simulink model "WT_GC"  (R2018a)
settings: Solver=ode5  StartTime=0.0  StopTime=8  FixedStep=Ts_phy  RelTol=1e-3  EnableMultiTasking=on
values from neighbouring files (symbols this model uses):
  col = {}    [Electrical_model_settings.m]    (also in WT_GC_Script.m)
  systemBase = {}    [Electrical_model_settings.m]    (also in WT_GC_Script.m)
  Ts_phy = 1/10000    (= 0.0001)    [Electrical_model_settings.m]    (also in WT_GC_Script.m)
  Ts_sim = Ts_phy    (= 0.0001)    [WT_GC_Script.m]
  wt1 = {}    [Electrical_model_settings.m]    (also in WT_GC_Script.m)
undefined symbols (not defined in the file or in its folder): D1, Delta
libraries: pwrsysBasic x42, powerlib x16, pwrsysVICtrl x12, pwrsysVSrc x3, pwrsysTransf x3, pwrsysVSrc_202301 x2
settings Model: Creator=daniemot  LastModifiedBy=daniemot
settings OptimizationCC: LifeSpan=inf
settings DebuggingCC: SFUnexpectedBacktrackingDiag=warning  SFNoUnconditionalDefaultTransitionDiag=warning  SFExecutionAtInitializationDiag=none
settings CodeAppCC: StateflowObjectComments=on
settings GRTTargetCC: TargetLangStandard=C89/C90 (ANSI)  GeneratePreprocessorConditionals=Disable all
settings ConfigComp: CovMetricSettings=dw  CovHtmlReporting=on  CovSaveCumulativeToWorkspaceVar=on  CovSaveSingleToWorkspaceVar=on  CovExternalEMLEnable=off
settings SimscapeCC: SimscapeNormalizeSystem=off

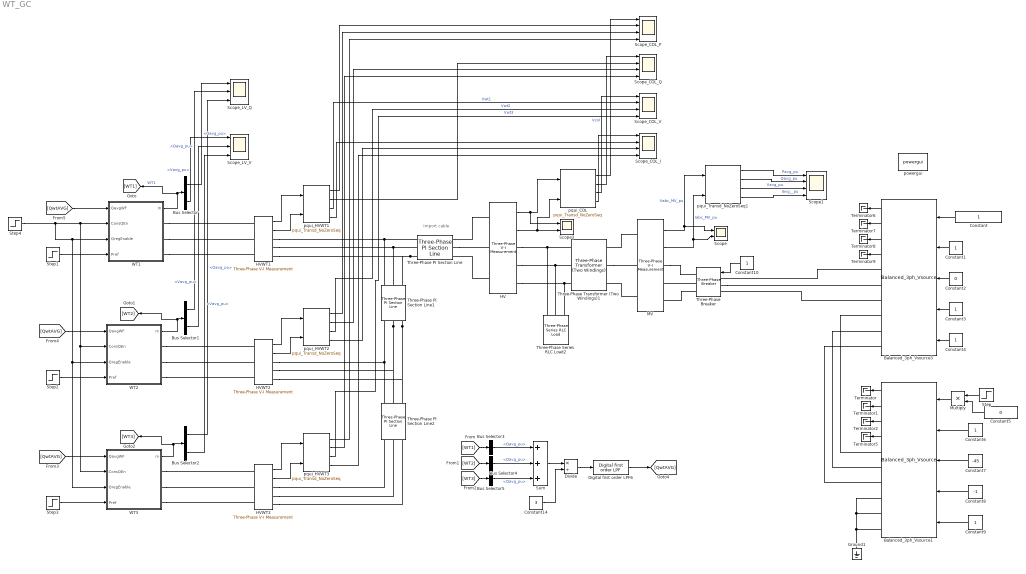
== system WT_GC ==
  note: Import cable
  Balanced_3ph_Vsource1 : pwrsysVSrc_202301/Balanced_3ph_Vsource  BaseAmp=sm.Vn_phase_peak  fn=sm.fn  AmpIni=0  SeqIni=-1  AngIni=0  FIni=sm.fn  HarmIni=1
  Balanced_3ph_Vsource3 : pwrsysVSrc_202301/Balanced_3ph_Vsource  BaseAmp=sm.Vn_phase_peak  fn=sm.fn  AmpIni=sm.Vn_phase_peak  SeqIni=1  AngIni=sm.phaseInitial  FIni=sm.initialSpeed  HarmIni=1
  Bus Selector : BusSelector  OutputSignals=Qavg_pu,Vavg_pu
  Bus Selector1 : BusSelector  OutputSignals=Qavg_pu,Vavg_pu
  Bus Selector2 : BusSelector  OutputSignals=Qavg_pu,Vavg_pu
  Bus Selector3 : BusSelector  OutputSignals=Qavg_pu
  Bus Selector4 : BusSelector  OutputSignals=Qavg_pu
  Bus Selector5 : BusSelector  OutputSignals=Qavg_pu
  Constant{,1,3..4,6,9..10} (7 alike) : Constant
  Constant14 : Constant  Value=3
  Constant2 : Constant  Value=0
  Constant5 : Constant  Value=0
  Constant7 : Constant  Value=-45
  Constant8 : Constant  Value=-1
  Digital first order LPF6 : pwrsysBasic/Digital first order LPF  Ts=wt1.Ts_control  fcutout=1
      settings: SourceProductName=NTNU Power Systems
  Divide : Product  Inputs=*/
  Ground1 : powerlib/Elements/Ground  LConnTagsString=a
  HV : powerlib/Measurements/Three-Phase V-I Measurement  VoltageMeasurement=phase-to-ground  SetLabelV=off  LabelV=vgrid  Vpu=off  VpuLL=off  CurrentMeasurement=yes  SetLabelI=off  LabelI=igrid  Ipu=off  Pbase=sn  Vbase=uab  OutputType=Complex  PhasorSimulation=off  PSBequivalent=0
  HVWT1 : powerlib/Measurements/Three-Phase V-I Measurement  VoltageMeasurement=phase-to-ground  SetLabelV=off  LabelV=vgrid  Vpu=off  VpuLL=off  CurrentMeasurement=yes  SetLabelI=off  LabelI=igrid  Ipu=off  Pbase=sn  Vbase=uab  OutputType=Complex  PhasorSimulation=off  PSBequivalent=0
  HVWT2 : powerlib/Measurements/Three-Phase V-I Measurement  VoltageMeasurement=phase-to-ground  SetLabelV=off  LabelV=vgrid  Vpu=off  VpuLL=off  CurrentMeasurement=yes  SetLabelI=off  LabelI=igrid  Ipu=off  Pbase=sn  Vbase=uab  OutputType=Complex  PhasorSimulation=off  PSBequivalent=0
  HVWT3 : powerlib/Measurements/Three-Phase V-I Measurement  VoltageMeasurement=phase-to-ground  SetLabelV=off  LabelV=vgrid  Vpu=off  VpuLL=off  CurrentMeasurement=yes  SetLabelI=off  LabelI=igrid  Ipu=off  Pbase=sn  Vbase=uab  OutputType=Complex  PhasorSimulation=off  PSBequivalent=0
  MV : powerlib/Measurements/Three-Phase V-I Measurement  VoltageMeasurement=phase-to-ground  SetLabelV=off  LabelV=vgrid  Vpu=off  VpuLL=off  CurrentMeasurement=yes  SetLabelI=off  LabelI=igrid  Ipu=off  Pbase=sn  Vbase=uab  OutputType=Complex  PhasorSimulation=off  PSBequivalent=0
  Multiply : Product
  Scope : Scope  NumInputPorts=2
  Scope1 : Scope  NumInputPorts=4
  Scope3 : Scope  NumInputPorts=2
  Scope_COL_I : Scope  NumInputPorts=4
  Scope_COL_P : Scope  NumInputPorts=4
  Scope_COL_Q : Scope  NumInputPorts=4
  Scope_COL_V : Scope  NumInputPorts=4
  Scope_LV_Q : Scope  NumInputPorts=3
  Scope_LV_V : Scope  NumInputPorts=3
  Step : Step  Time=0.1  SampleTime=0
  Step1 : Step  Time=wt1.DCVCont.Start+2.8  After=0.8  SampleTime=0
  Step2 : Step  Time=wt1.DCVCont.Start+1.8  After=0.8  SampleTime=0
  Step3 : Step  Time=wt1.DCVCont.Start+0.8  After=0.8  SampleTime=0
  Step4 : Step  Time=5  SampleTime=0
  Sum : Sum  Inputs=+++
  Terminator{,1..2,5..9} (8 alike) : Terminator
  Three-Phase PI Section Line : powerlib/Elements/Three-Phase PI Section Line  LConnTagsString=a|b|c  RConnTagsString=A|B|C  Frequency=systemBase.fn  Resistances=[ col.Cable.Rpos col.Cable.Rzero]  Inductances=[ col.Cable.Lpos col.Cable.Lzero]  Capacitances=[col.Cable.Cpos col.Cable.Czero]  Length=col.Cable.Limport
      settings: SourceProductName=Simscape Power Systems
  Three-Phase PI Section Line1 : powerlib/Elements/Three-Phase PI Section Line  LConnTagsString=a|b|c  RConnTagsString=A|B|C  Frequency=systemBase.fn  Resistances=[ col.Cable.Rpos col.Cable.Rzero]  Inductances=[ col.Cable.Lpos col.Cable.Lzero]  Capacitances=[col.Cable.Cpos col.Cable.Czero]  Length=col.Cable.LinterWT
      settings: SourceProductName=Simscape Power Systems
  Three-Phase PI Section Line2 : powerlib/Elements/Three-Phase PI Section Line  LConnTagsString=a|b|c  RConnTagsString=A|B|C  Frequency=systemBase.fn  Resistances=[ col.Cable.Rpos col.Cable.Rzero]  Inductances=[ col.Cable.Lpos col.Cable.Lzero]  Capacitances=[col.Cable.Cpos col.Cable.Czero]  Length=col.Cable.LinterWT
      settings: SourceProductName=Simscape Power Systems
  Three-Phase Series RLC Load2 : powerlib/Elements/Three-Phase Series RLC Load  LConnTagsString=A|B|C  Configuration=Y (grounded)  NominalVoltage=systemBase.Vn  Vabc=[1e3 1e3 1e3]  Vabcp=[1e3 1e3 1e3]  NominalFrequency=systemBase.fn  UnbalancedPower=off  ActivePower=100  InductivePower=0  CapacitivePower=0  Pabc=[10e3 9e3 11e3]  QLabc=[100 90 110]  QCabc=[100 90 110]  Pabcp=[10e3 9e3 11e3]  QLabcp=[100 90 110]  QCabcp=[100 90 110]  Measurements=None  LoadType=constant Z
  Three-Phase Transformer (Two Windings)1 : powerlib/Elements/Three-Phase Transformer (Two Windings)  Winding1Connection=Delta (D1)  Winding2Connection=Y  CoreType=Three-limb core (core-type)  SetSaturation=off  Hysteresis=off  DataFile='hysteresis'  SetInitialFlux=off  Measurements=None  UNITS=pu  NominalPower=[ col.Sn , systemBase.fn ]  Winding1=[ systemBase.Vn , col.Trafo.rsc/2 , col.Trafo.xsc/2 ]  Winding2=[ col.Un , col.Trafo.rsc/2 , col.Trafo.xsc/2 ]  Rm=500  Lm=500  L0=0.5  Saturation=[ 0,0 ; 0.0024,1.2 ; 1.0,1.52 ]  InitialFluxes=[ 0.8 , -0.8 , 0.7 ]  MoreParameters=off  BreakLoop=off  DataType=off  TransfoNumber=1
  Three-Phase Breaker : powerlib/Elements/Three-Phase Breaker  InitialState=closed  SwitchA=on  SwitchB=on  SwitchC=on  SwitchTimes="[1/60  5/60]"  External=on  BreakerResistance=0.01  SnubberResistance=1e6  SnubberCapacitance=1e9  Measurements=None
  WT1 : Subsystem
  WT2 : Subsystem
  WT3 : Subsystem
  powergui : powerlib/powergui  Priority=1  SimulationMode=Discrete  SampleTime=max(Ts_phy,Ts_sim)  frequency=60  Iterations=50  frequencyindice=0  Pbase=100e6  ErrMax=1e-4  UnitsV=kV  UnitsW=MW  buscounter=0  FunctionMessages=off  echomessages=off  EnableUseOfTLC=off  CurrentSourceSwitches=off  DisableSnubberDevices=off  DisableRonSwitches=off  DisableVfSwitches=off  DisplayEquations=off  SolverType=Tustin/Backward Euler (TBE)  Interpol=off  ExternalGateDelay=off  methode=off  Ts=100  x0status=blocks  SPID=off  SwTol=0  HookPort=off  RestoreLinks=warning  ResistiveCurrentMeasurement=off  Frange=[0:2:500]  Ylog=off  Xlog=on  ShowGrid=off  save=off  variable=ZData  structure=0  ZoomFFT=off  StartTime=0.0  cycles=1  DisplayStyle=1  fundamental=60  FreqAxis=off  MaxFrequency=1000  frequencyindicesteady=1  RmsSteady=1  display=off
  pqui_COL : pwrsysBasic/pqui_Transd_NoZeroSeq  Sn=col.Sn  Uanp=col.Uanp  Iap=col.Iap
      settings: SourceProductName=NTNU Power Systems
  pqui_HVWT1 : pwrsysBasic/pqui_Transd_NoZeroSeq  Sn=wt1.Sn  Uanp=col.Uanp  Iap=wt1.Iap*(wt1.Un/col.Un)
      settings: SourceProductName=NTNU Power Systems
  pqui_HVWT2 : pwrsysBasic/pqui_Transd_NoZeroSeq  Sn=wt1.Sn  Uanp=col.Uanp  Iap=wt1.Iap*(wt1.Un/col.Un)
      settings: SourceProductName=NTNU Power Systems
  pqui_HVWT3 : pwrsysBasic/pqui_Transd_NoZeroSeq  Sn=wt1.Sn  Uanp=col.Uanp  Iap=wt1.Iap*(wt1.Un/col.Un)
      settings: SourceProductName=NTNU Power Systems
  pqui_Transd_NoZeroSeq1 : pwrsysBasic/pqui_Transd_NoZeroSeq  Sn=col.Sn  Uanp=systemBase.Vn_phase*sqrt(2)  Iap=col.Iap*(col.Un/systemBase.Vn_phase)
      settings: SourceProductName=NTNU Power Systems
  wires:
  Constant/1 -> Balanced_3ph_Vsource3/1
  Balanced_3ph_Vsource3/3 -> Terminator8/1
  Balanced_3ph_Vsource1/4 -> Terminator5/1
  Step/1 -> Multiply/1
  Balanced_3ph_Vsource3/4 -> Terminator9/1
  Balanced_3ph_Vsource3/1 -> Terminator6/1
  Balanced_3ph_Vsource1/3 -> Terminator2/1
  Balanced_3ph_Vsource3/2 -> Terminator7/1
  Constant9/1 -> Balanced_3ph_Vsource1/5
  Constant2/1 -> Balanced_3ph_Vsource3/3
  Constant7/1 -> Balanced_3ph_Vsource1/3
  Constant5/1 -> Multiply/2
  Multiply/1 -> Balanced_3ph_Vsource1/1
  Constant8/1 -> Balanced_3ph_Vsource1/4
  Balanced_3ph_Vsource1/1 -> Terminator/1
  Balanced_3ph_Vsource1/2 -> Terminator1/1
  Constant3/1 -> Balanced_3ph_Vsource3/4
  Constant6/1 -> Balanced_3ph_Vsource1/2
  Constant4/1 -> Balanced_3ph_Vsource3/5
  Constant1/1 -> Balanced_3ph_Vsource3/2
  Constant10/1 -> Three-Phase Breaker/1
  MV/2 -> Scope/2, pqui_Transd_NoZeroSeq1/2  "Iabc_MV_pu"
  pqui_Transd_NoZeroSeq1/1 -> Scope1/1  "Pavg_pu"
  MV/1 -> Scope/1, pqui_Transd_NoZeroSeq1/1  "Vabc_MV_pu"
  pqui_Transd_NoZeroSeq1/3 -> Scope1/3  "Vavg_pu"
  pqui_Transd_NoZeroSeq1/2 -> Scope1/2  "Qavg_pu"
  pqui_Transd_NoZeroSeq1/4 -> Scope1/4  "Iavg__pu"
  [QwtAVG] -> WT1/1(QavgWF)
  HV/1 -> Scope3/1, pqui_COL/1
  HV/2 -> Scope3/2, pqui_COL/2
  pqui_COL/1 -> Scope_COL_P/1
  pqui_COL/2 -> Scope_COL_Q/1
  pqui_COL/3 -> Scope_COL_V/1  "Vcol"
  Step1/1 -> WT1/4(Pref)
  WT2/1(m) -> [WT2], Bus Selector1/1
  WT3/1(m) -> [WT3], Bus Selector2/1
  WT1/1(m) -> [WT1], Bus Selector/1  "WT1"
  HVWT1/2 -> pqui_HVWT1/2
  HVWT1/1 -> pqui_HVWT1/1
  pqui_HVWT1/3 -> Scope_COL_V/2  "Vwt1"
  HVWT2/1 -> pqui_HVWT2/1
  HVWT2/2 -> pqui_HVWT2/2
  HVWT3/1 -> pqui_HVWT3/1
  HVWT3/2 -> pqui_HVWT3/2
  pqui_HVWT3/3 -> Scope_COL_V/4  "Vwt3"
  pqui_HVWT2/3 -> Scope_COL_V/3  "Vwt2"
  pqui_HVWT1/2 -> Scope_COL_Q/2
  pqui_HVWT2/2 -> Scope_COL_Q/3
  pqui_HVWT3/2 -> Scope_COL_Q/4
  pqui_HVWT1/1 -> Scope_COL_P/2
  pqui_HVWT2/1 -> Scope_COL_P/3
  pqui_HVWT3/1 -> Scope_COL_P/4
  pqui_COL/4 -> Scope_COL_I/1
  pqui_HVWT1/4 -> Scope_COL_I/2
  pqui_HVWT2/4 -> Scope_COL_I/3
  pqui_HVWT3/4 -> Scope_COL_I/4
  Bus Selector/1 -> Scope_LV_Q/1  "<Qavg_pu>"
  Bus Selector1/1 -> Scope_LV_Q/2  "<Qavg_pu>"
  Bus Selector2/1 -> Scope_LV_Q/3  "<Qavg_pu>"
  Bus Selector/2 -> Scope_LV_V/1  "<Vavg_pu>"
  Bus Selector1/2 -> Scope_LV_V/2  "<Vavg_pu>"
  Bus Selector2/2 -> Scope_LV_V/3  "<Vavg_pu>"
  Step4/1 -> WT2/3(QregEnable), WT3/3(QregEnable), WT1/3(QregEnable), WT3/2(ConsQEn), WT2/2(ConsQEn), WT1/2(ConsQEn)
  Step2/1 -> WT2/4(Pref)
  Step3/1 -> WT3/4(Pref)
  [WT1] -> Bus Selector3/1
  [WT2] -> Bus Selector4/1
  [WT3] -> Bus Selector5/1
  Bus Selector3/1 -> Sum/1  "<Qavg_pu>"
  Bus Selector4/1 -> Sum/2  "<Qavg_pu>"
  Bus Selector5/1 -> Sum/3  "<Qavg_pu>"
  Sum/1 -> Divide/1
  Constant14/1 -> Divide/2
  Divide/1 -> Digital first order LPF6/1
  Digital first order LPF6/1 -> [QwtAVG]
  [QwtAVG] -> WT3/1(QavgWF)
  [QwtAVG] -> WT2/1(QavgWF)
  connections:
  Balanced_3ph_Vsource1/RConn4 -- Balanced_3ph_Vsource1/RConn6 -- Ground1/LConn1 -- Balanced_3ph_Vsource1/RConn5
  Balanced_3ph_Vsource1/RConn1 -- Balanced_3ph_Vsource3/RConn4
  Balanced_3ph_Vsource1/RConn2 -- Balanced_3ph_Vsource3/RConn5
  Balanced_3ph_Vsource1/RConn3 -- Balanced_3ph_Vsource3/RConn6
  MV/RConn1 -- Three-Phase Breaker/RConn1
  Three-Phase Breaker/RConn2 -- MV/RConn2
  Three-Phase Breaker/RConn3 -- MV/RConn3
  Three-Phase Breaker/LConn2 -- Balanced_3ph_Vsource3/RConn2
  Balanced_3ph_Vsource3/RConn1 -- Three-Phase Breaker/LConn1
  Balanced_3ph_Vsource3/RConn3 -- Three-Phase Breaker/LConn3
  Three-Phase Transformer (Two Windings)1/LConn2 -- MV/LConn2
  MV/LConn1 -- Three-Phase Transformer (Two Windings)1/LConn1
  MV/LConn3 -- Three-Phase Transformer (Two Windings)1/LConn3
  Three-Phase Series RLC Load2/LConn1 -- HV/RConn1 -- Three-Phase Transformer (Two Windings)1/RConn1
  Three-Phase Transformer (Two Windings)1/RConn2 -- HV/RConn2 -- Three-Phase Series RLC Load2/LConn2
  Three-Phase Transformer (Two Windings)1/RConn3 -- HV/RConn3 -- Three-Phase Series RLC Load2/LConn3
  Three-Phase PI Section Line1/LConn1 -- HVWT1/RConn1 -- Three-Phase PI Section Line/LConn1
  Three-Phase PI Section Line/LConn3 -- HVWT1/RConn3 -- Three-Phase PI Section Line1/LConn3
  Three-Phase PI Section Line1/LConn2 -- HVWT1/RConn2 -- Three-Phase PI Section Line/LConn2
  HV/LConn1 -- Three-Phase PI Section Line/RConn1
  Three-Phase PI Section Line/RConn2 -- HV/LConn2
  HV/LConn3 -- Three-Phase PI Section Line/RConn3
  Three-Phase PI Section Line2/LConn1 -- HVWT2/RConn1 -- Three-Phase PI Section Line1/RConn1
  Three-Phase PI Section Line1/RConn2 -- Three-Phase PI Section Line2/LConn2 -- HVWT2/RConn2
  Three-Phase PI Section Line1/RConn3 -- Three-Phase PI Section Line2/LConn3 -- HVWT2/RConn3
  WT1/RConn1 -- HVWT1/LConn1
  WT1/RConn2 -- HVWT1/LConn2
  WT1/RConn3 -- HVWT1/LConn3
  WT2/RConn1 -- HVWT2/LConn1
  WT2/RConn2 -- HVWT2/LConn2
  WT2/RConn3 -- HVWT2/LConn3
  WT3/RConn1 -- HVWT3/LConn1
  WT3/RConn2 -- HVWT3/LConn2
  WT3/RConn3 -- HVWT3/LConn3
  HVWT3/RConn1 -- Three-Phase PI Section Line2/RConn1
  HVWT3/RConn2 -- Three-Phase PI Section Line2/RConn2
  HVWT3/RConn3 -- Three-Phase PI Section Line2/RConn3

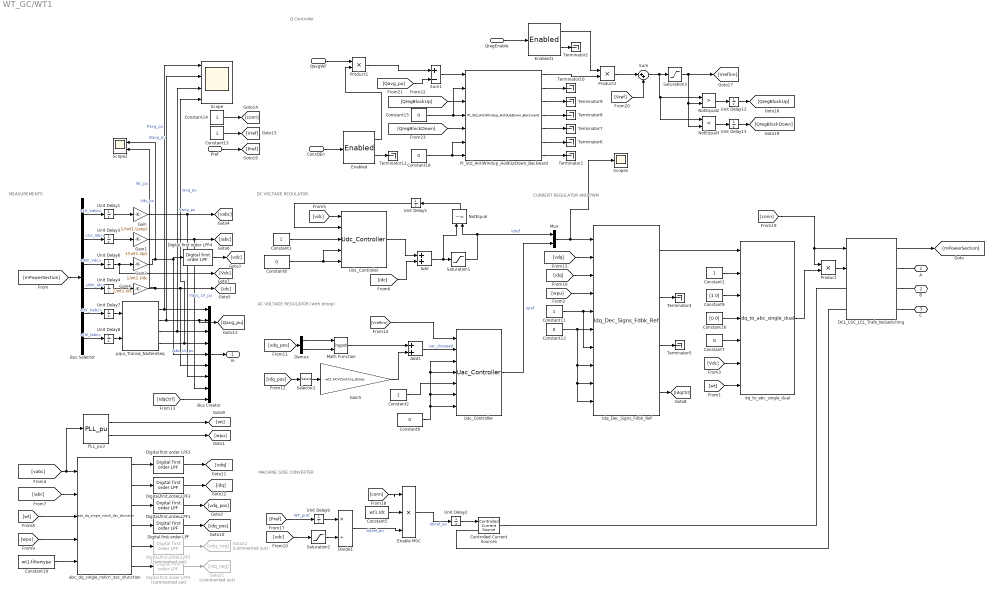
== system WT_GC/WT1 ==
  note: MEASUREMENTS
  note: MACHINE SIDE CONVERTER
  note: AC VOLTAGE REGULATOR (with droop)
  note: DC VOLTAGE REGULATOR
  note: CURRENT REGULATOR AND PWM
  note: Q Controller
  QavgWF : Inport
  ConsQEn : Inport  Port=2
  QregEnable : Inport  Port=3
  Pref : Inport  Port=4
  Add : Sum
  Add1 : Sum
  Bus Creator : BusCreator  Inputs=9
  Bus Selector : BusSelector  OutputSignals=LV_Vabc,LV_Iabc,INV_Vdc,INV_Idc,HV_Vabc,HV_Iabc
  Constant{1..3,11} (4 alike) : Constant  SampleTime=wt1.Ts_control
  Constant10 : Constant  Value=wt1.filtertype  SampleTime=wt1.Ts_control
  Constant{6..8,12} (4 alike) : Constant  Value=0  SampleTime=wt1.Ts_control
  Constant13 : Constant
  Constant14 : Constant
  Constant15 : Constant  Value=0
  Constant16 : Constant  Value=[0 0]  SampleTime=wt1.Ts_control
  Constant18 : Constant  Value=0
  Constant5 : Constant  Value=wt1.Idc  SampleTime=wt1.Ts_control
  Constant9 : Constant  Value=[1 0]  SampleTime=wt1.Ts_control
  Controlled Current Source1 : powerlib/Electrical Sources/Controlled Current Source  Initialize=on  Source_Type=DC  Amplitude=0  Phase=0  Frequency=50  Measurements=None
  DCL_LSC_LCL_Trafo_NoSwitching : pwrsysVSrc/DCL_LSC_LCL_Trafo_NoSwitching  Sn=wt1.Sn  fn=systemBase.fn  Uhv_ab=col.Un  Uab=wt1.Un  lf2=wt1.LCL.l2  rf2=wt1.LCL.r2  Lf1=wt1.LCL.L1  Rf1=wt1.LCL.R1  Cf=wt1.LCL.Cf  Rc=wt1.LCL.Rf  Cdc=wt1.Cdc  Udc0=wt1.Udc  Tsm=wt1.Ts_control  Tstart=wt1.DCVCont.Start
      settings: SourceProductName=NTNU Power Systems
  Demux : Demux  Outputs=2
  Digital first order LPF{,1..4} (5 alike) : pwrsysBasic/Digital first order LPF  Ts=wt1.Ts_control  fcutout=wt1.CurrCont.f_LPF_noise
      settings: SourceProductName=NTNU Power Systems
  Digital first order LPF5 : pwrsysBasic/Digital first order LPF  Commented=on  Ts=wt1.Ts_control  fcutout=wt1.CurrCont.f_LPF_noise
      settings: SourceProductName=NTNU Power Systems
  Digital first order LPF6 : pwrsysBasic/Digital first order LPF  Commented=on  Ts=wt1.Ts_control  fcutout=wt1.CurrCont.f_LPF_noise
      settings: SourceProductName=NTNU Power Systems
  Divide1 : Product  Inputs=*/
  Enable MSC : Product  Inputs=3
  Enabled : pwrsysBasic/Enabled
      settings: SourceProductName=NTNU Power Systems
  Enabled1 : pwrsysBasic/Enabled
      settings: SourceProductName=NTNU Power Systems
  Gain : Gain  Gain=1/(wt1.Uanp)
  Gain1 : Gain  Gain=1/(wt1.Iap)
  Gain2 : Gain  Gain=1/wt1.Udc
  Gain4 : Gain  Gain=1/wt1.Idc
  Gain5 : Gain  Gain=-wt1.ACVCont.kiq_droop
  Goto21 : Goto  Commented=on  GotoTag=idq_neg
  Goto22 : Goto  Commented=on  GotoTag=vdq_neg
  Idq_Dec_Signs_Fdbk_Ref : pwrsysVICtrl/Idq_Dec_Signs_Fdbk_Ref  Ts=wt1.Ts_control  fn=systemBase.fn  Kp=wt1.CurrContSingle.kp  Ti=wt1.CurrContSingle.Ti  L=wt1.CurrCont.x  PI_max=wt1.CurrCont.PImax  PI_min=wt1.CurrCont.PImin  TrafoPhaseComp=0
      settings: SourceProductName=NTNU Power Systems
  Math Function : Math  Operator=hypot  SaturateOnIntegerOverflow=on
  Mux : Mux  Inputs=2
  NotEqual : RelationalOperator  Operator=~=  OutDataTypeStr=boolean  RndMeth=Nearest
  NotEqual2 : RelationalOperator  Operator=>  OutDataTypeStr=boolean  RndMeth=Nearest
  NotEqual3 : RelationalOperator  Operator=<  OutDataTypeStr=boolean  RndMeth=Nearest
  PI_Std_AntiWindup_HoldUpDown_Backward : pwrsysBasic/PI_Std_AntiWindup_HoldUpDown_Backward  Ts=wt1.Ts_control  Kg=wt1.Qctrl.Kg  Kp=wt1.Qctrl.Kp  Ti=wt1.Qctrl.Ti  outMax=wt1.Qctrl.deltaUmaxPos  outMin=wt1.Qctrl.deltaUmaxNeg
      settings: SourceProductName=NTNU Power Systems
  PLL_pu3 : pwrsysBasic/PLL_pu  fn=systemBase.fn  Ts=wt1.Ts_control  Kp_pll=90  Ki_pll=1200  Kd_pll=0  PLL_ini=60
      settings: SourceProductName=NTNU Power Systems
  Product : Product
  Product1 : Product
  Product2 : Product
  Saturation1 : Saturate  UpperLimit=wt1.DCVCont.PImax  LowerLimit=wt1.DCVCont.PImin
  Saturation2 : Saturate  UpperLimit=1.2  LowerLimit=0.8
  Saturation3 : Saturate  UpperLimit=wt1.Qctrl.Umax  LowerLimit=wt1.Qctrl.Umin
  Scope : Scope  NumInputPorts=4
  Scope1 : Scope
  Scope2 : Scope  NumInputPorts=2
  Selector2 : Selector  IndexMode=Zero-based  InputPortWidth=2  IndexOptions=Index vector (dialog)  Indices=1  OutputSizes=1
  Sum : Sum  Inputs=|++
  Sum1 : Sum  Inputs=+-
  Terminator{1..2,4..10,12} (10 alike) : Terminator
  Uac_Controller : pwrsysVICtrl/Uac_Controller  Ts=wt1.Ts_control  Kg=wt1.ACVCont.kg  Kp=wt1.ACVCont.kp  Ti=wt1.ACVCont.Ti  PI_max=wt1.ACVCont.PImax  PI_min=wt1.ACVCont.PImin
      settings: SourceProductName=NTNU Power Systems
  Udc_Controller : pwrsysVICtrl/Udc_Controller  Ts=wt1.Ts_control  Kp=wt1.DCVContSingle.kp  Ti=wt1.DCVContSingle.Ti  PI_max=wt1.DCVCont.PImax  PI_min=wt1.DCVCont.PImin
      settings: SourceProductName=NTNU Power Systems
  Unit Delay{1,3,7..8} (4 alike) : UnitDelay  InitialCondition=[0 0 0]  SampleTime=wt1.Ts_control
  Unit Delay{2,4..5,9,12..13} (6 alike) : UnitDelay  SampleTime=wt1.Ts_control
  Unit Delay6 : UnitDelay  InitialCondition=1  SampleTime=wt1.Ts_control
  abc_dq_single_notch_dsc_sfunction : pwrsysTransf/abc_dq_single_notch_dsc_sfunction  Ts=wt1.Ts_control  fn=2*systemBase.fn  zeta=wt1.CurrCont.zeta
      settings: SourceProductName=NTNU Power Systems
  dq_to_abc_single_dual : pwrsysVICtrl/dq_to_abc_single_dual  Ts=wt1.Ts_control  Uabp=wt1.Uabp
      settings: SourceProductName=NTNU Power Systems
  pqui_Transd_NoZeroSeq : pwrsysBasic/pqui_Transd_NoZeroSeq  Sn=wt1.Sn  Uanp=col.Uanp  Iap=wt1.Iap*(wt1.Un/col.Un)
      settings: SourceProductName=NTNU Power Systems
  A : PMIOPort  Side=Right
  B : PMIOPort  Port=2  Side=Right
  C : PMIOPort  Port=3  Side=Right
  m : Outport
  wires:
  Divide1/1 -> Enable MSC/3  "Idcref_pu"
  Bus Selector/1 -> Unit Delay1/1  "<LV_Vabc>"
  [idq_pos] -> Selector2/1
  Unit Delay2/1 -> Controlled Current Source1/1
  Gain1/1 -> Bus Creator/8, [iabc]  "Iabc_LV_pu"
  Bus Selector/2 -> Unit Delay3/1  "<LV_Iabc>"
  Gain5/1 -> Add1/2
  Math Function/1 -> Add1/1
  Constant6/1 -> Uac_Controller/7, Uac_Controller/6, Uac_Controller/3, Uac_Controller/4
  Constant5/1 -> Enable MSC/2
  Add1/1 -> Uac_Controller/2  "vac_drooped"
  [mPowerSection] -> Bus Selector/1
  Enable MSC/1 -> Unit Delay2/1  "Idcref_pu"
  Gain/1 -> Bus Creator/7, [vabc]  "Vabc_LV_pu"
  Constant2/1 -> Uac_Controller/5
  Constant8/1 -> Udc_Controller/4, Udc_Controller/5
  NotEqual/1 -> Unit Delay5/1
  [vdc] -> Udc_Controller/1
  Unit Delay5/1 -> Udc_Controller/2
  Saturation1/1 -> NotEqual/2, Mux/1  "idref"
  [idc] -> Add/2
  Udc_Controller/1 -> Add/1
  Add/1 -> NotEqual/1, Saturation1/1
  Constant3/1 -> Udc_Controller/3
  [idq] -> Idq_Dec_Signs_Fdbk_Ref/3
  [Vdc] -> dq_to_abc_single_dual/6
  [wpu] -> Idq_Dec_Signs_Fdbk_Ref/4
  dq_to_abc_single_dual/1 -> Product/2
  [conn] -> Product/1, DCL_LSC_LCL_Trafo_NoSwitching/1
  Saturation2/1 -> Divide1/2
  [Pref] -> Unit Delay9/1  "WT_pref"
  [vdc] -> Saturation2/1
  [wt] -> dq_to_abc_single_dual/7
  Constant10/1 -> abc_dq_single_notch_dsc_sfunction/5
  Bus Selector/5 -> Unit Delay7/1  "<HV_Vabc>"
  Bus Selector/6 -> Unit Delay8/1  "<HV_Iabc>"
  pqui_Transd_NoZeroSeq/1 -> Scope/1, Bus Creator/1  "Pavg_pu"
  pqui_Transd_NoZeroSeq/2 -> Scope/2, [Qavg_pu], Bus Creator/2  "Qavg_pu"
  pqui_Transd_NoZeroSeq/3 -> Scope/3, Bus Creator/3  "Vavg_pu"
  pqui_Transd_NoZeroSeq/4 -> Scope/4, Bus Creator/4  "Iavg_pu"
  Bus Creator/1 -> m/1
  Bus Selector/3 -> Unit Delay6/1  "<INV_Vdc>"
  Gain2/1 -> Scope2/1, Digital first order LPF4/1, Bus Creator/5  "Vdc_pu"
  Gain4/1 -> Scope2/2, [idc], Bus Creator/6  "Idc_pu"
  Bus Selector/4 -> Unit Delay4/1  "<INV_Idc>"
  PLL_pu3/2 -> [wpu]
  PLL_pu3/1 -> [wt]
  Uac_Controller/1 -> Mux/2  "iqref"
  DCL_LSC_LCL_Trafo_NoSwitching/1 -> [mPowerSection]
  Unit Delay1/1 -> Gain/1
  Unit Delay3/1 -> Gain1/1
  Unit Delay4/1 -> Gain4/1
  Unit Delay8/1 -> pqui_Transd_NoZeroSeq/2
  Unit Delay6/1 -> [Vdc], Gain2/1
  Unit Delay7/1 -> pqui_Transd_NoZeroSeq/1
  Unit Delay9/1 -> Divide1/1
  [Vreflim] -> Uac_Controller/1
  abc_dq_single_notch_dsc_sfunction/6 -> Digital first order LPF6/1
  abc_dq_single_notch_dsc_sfunction/5 -> Digital first order LPF5/1
  Selector2/1 -> Gain5/1
  Idq_Dec_Signs_Fdbk_Ref/2 -> Terminator4/1
  [vdq] -> Idq_Dec_Signs_Fdbk_Ref/2
  Constant1/1 -> dq_to_abc_single_dual/2
  Constant7/1 -> dq_to_abc_single_dual/5
  Constant11/1 -> Idq_Dec_Signs_Fdbk_Ref/7, Idq_Dec_Signs_Fdbk_Ref/5
  Constant12/1 -> Idq_Dec_Signs_Fdbk_Ref/8, Idq_Dec_Signs_Fdbk_Ref/9, Idq_Dec_Signs_Fdbk_Ref/10, Idq_Dec_Signs_Fdbk_Ref/6
  Idq_Dec_Signs_Fdbk_Ref/3 -> Terminator5/1
  Idq_Dec_Signs_Fdbk_Ref/4 -> [IdqCtrl]
  [IdqCtrl] -> Bus Creator/9
  Idq_Dec_Signs_Fdbk_Ref/1 -> dq_to_abc_single_dual/1
  [wt] -> abc_dq_single_notch_dsc_sfunction/3
  [wpu] -> abc_dq_single_notch_dsc_sfunction/4
  abc_dq_single_notch_dsc_sfunction/1 -> Digital first order LPF2/1
  [vabc] -> abc_dq_single_notch_dsc_sfunction/1, PLL_pu3/1
  [iabc] -> abc_dq_single_notch_dsc_sfunction/2
  abc_dq_single_notch_dsc_sfunction/3 -> Digital first order LPF1/1
  abc_dq_single_notch_dsc_sfunction/4 -> Digital first order LPF/1
  abc_dq_single_notch_dsc_sfunction/2 -> Digital first order LPF3/1
  Digital first order LPF/1 -> [idq_pos]
  Digital first order LPF1/1 -> [vdq_pos]
  [vdq_pos] -> Demux/1
  Demux/1 -> Math Function/1
  Demux/2 -> Math Function/2
  Digital first order LPF2/1 -> [vdq]
  Digital first order LPF3/1 -> [idq]
  Digital first order LPF4/1 -> [vdc]
  [conn] -> Enable MSC/1
  Pref/1 -> [Pref]
  Mux/1 -> Scope1/1, Idq_Dec_Signs_Fdbk_Ref/1
  Product/1 -> DCL_LSC_LCL_Trafo_NoSwitching/2
  [Vref] -> Sum/2
  Sum/1 -> NotEqual3/1, NotEqual2/1, Saturation3/1
  Saturation3/1 -> NotEqual3/2, NotEqual2/2, [Vreflim]
  [Qavg_pu] -> Sum1/2
  ConsQEn/1 -> Enabled/1
  [QregBlockUp] -> PI_Std_AntiWindup_HoldUpDown_Backward/3
  Constant15/1 -> PI_Std_AntiWindup_HoldUpDown_Backward/2, PI_Std_AntiWindup_HoldUpDown_Backward/4
  [QregBlockDown] -> PI_Std_AntiWindup_HoldUpDown_Backward/5
  Constant18/1 -> PI_Std_AntiWindup_HoldUpDown_Backward/6, PI_Std_AntiWindup_HoldUpDown_Backward/7
  PI_Std_AntiWindup_HoldUpDown_Backward/7 -> Terminator1/1
  PI_Std_AntiWindup_HoldUpDown_Backward/6 -> Terminator6/1
  PI_Std_AntiWindup_HoldUpDown_Backward/5 -> Terminator7/1
  PI_Std_AntiWindup_HoldUpDown_Backward/4 -> Terminator8/1
  PI_Std_AntiWindup_HoldUpDown_Backward/3 -> Terminator9/1
  PI_Std_AntiWindup_HoldUpDown_Backward/2 -> Terminator10/1
  NotEqual2/1 -> Unit Delay12/1
  Unit Delay12/1 -> [QregBlockUp]
  NotEqual3/1 -> Unit Delay13/1
  Unit Delay13/1 -> [QregBlockDown]
  Product2/1 -> Sum/1
  Sum1/1 -> PI_Std_AntiWindup_HoldUpDown_Backward/1
  Enabled/2 -> Terminator12/1
  QavgWF/1 -> Product1/1
  Product1/1 -> Sum1/1
  Enabled/1 -> Product1/2
  Constant13/1 -> [Vref]
  Constant14/1 -> [conn]
  Digital first order LPF5/1 -> Goto22/1
  Digital first order LPF6/1 -> Goto21/1
  Constant9/1 -> dq_to_abc_single_dual/3
  Constant16/1 -> dq_to_abc_single_dual/4
  Enabled1/2 -> Terminator2/1
  PI_Std_AntiWindup_HoldUpDown_Backward/1 -> Product2/2
  Enabled1/1 -> Product2/1
  QregEnable/1 -> Enabled1/1
  connections:
  Controlled Current Source1/RConn1 -- DCL_LSC_LCL_Trafo_NoSwitching/LConn1
  DCL_LSC_LCL_Trafo_NoSwitching/RConn3 -- C/RConn1
  DCL_LSC_LCL_Trafo_NoSwitching/RConn1 -- A/RConn1
  DCL_LSC_LCL_Trafo_NoSwitching/RConn2 -- B/RConn1
  Controlled Current Source1/LConn1 -- DCL_LSC_LCL_Trafo_NoSwitching/LConn2

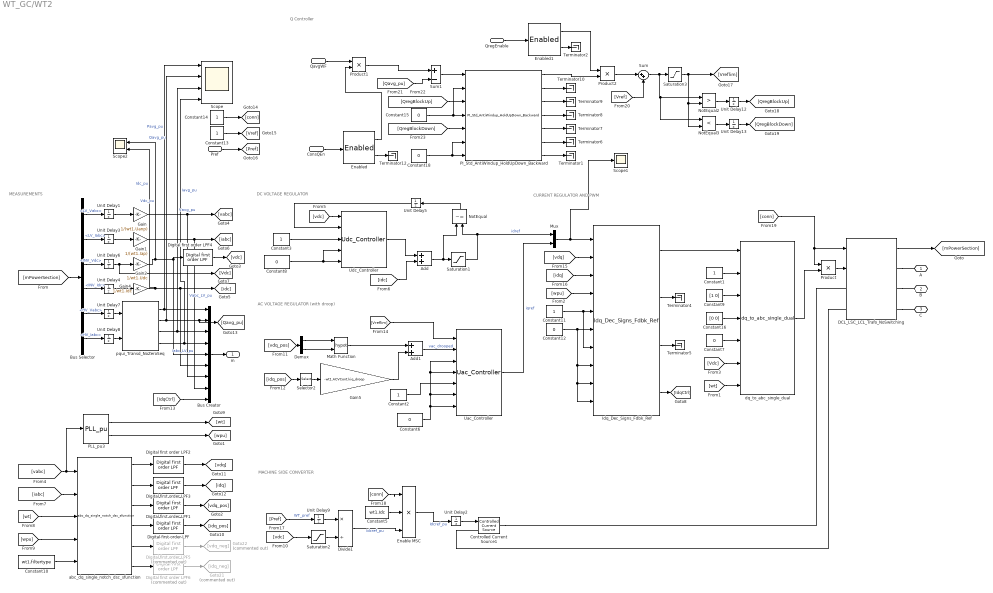
== system WT_GC/WT2 ==
  note: MEASUREMENTS
  note: MACHINE SIDE CONVERTER
  note: AC VOLTAGE REGULATOR (with droop)
  note: DC VOLTAGE REGULATOR
  note: CURRENT REGULATOR AND PWM
  note: Q Controller
  QavgWF : Inport
  ConsQEn : Inport  Port=2
  QregEnable : Inport  Port=3
  Pref : Inport  Port=4
  Add : Sum
  Add1 : Sum
  Bus Creator : BusCreator  Inputs=9
  Bus Selector : BusSelector  OutputSignals=LV_Vabc,LV_Iabc,INV_Vdc,INV_Idc,HV_Vabc,HV_Iabc
  Constant{1..3,11} (4 alike) : Constant  SampleTime=wt1.Ts_control
  Constant10 : Constant  Value=wt1.filtertype  SampleTime=wt1.Ts_control
  Constant{6..8,12} (4 alike) : Constant  Value=0  SampleTime=wt1.Ts_control
  Constant13 : Constant
  Constant14 : Constant
  Constant15 : Constant  Value=0
  Constant16 : Constant  Value=[0 0]  SampleTime=wt1.Ts_control
  Constant18 : Constant  Value=0
  Constant5 : Constant  Value=wt1.Idc  SampleTime=wt1.Ts_control
  Constant9 : Constant  Value=[1 0]  SampleTime=wt1.Ts_control
  Controlled Current Source1 : powerlib/Electrical Sources/Controlled Current Source  Initialize=on  Source_Type=DC  Amplitude=0  Phase=0  Frequency=50  Measurements=None
  DCL_LSC_LCL_Trafo_NoSwitching : pwrsysVSrc/DCL_LSC_LCL_Trafo_NoSwitching  Sn=wt1.Sn  fn=systemBase.fn  Uhv_ab=col.Un  Uab=wt1.Un  lf2=wt1.LCL.l2  rf2=wt1.LCL.r2  Lf1=wt1.LCL.L1  Rf1=wt1.LCL.R1  Cf=wt1.LCL.Cf  Rc=wt1.LCL.Rf  Cdc=wt1.Cdc  Udc0=wt1.Udc  Tsm=wt1.Ts_control  Tstart=wt1.DCVCont.Start
      settings: SourceProductName=NTNU Power Systems
  Demux : Demux  Outputs=2
  Digital first order LPF{,1..4} (5 alike) : pwrsysBasic/Digital first order LPF  Ts=wt1.Ts_control  fcutout=wt1.CurrCont.f_LPF_noise
      settings: SourceProductName=NTNU Power Systems
  Digital first order LPF5 : pwrsysBasic/Digital first order LPF  Commented=on  Ts=wt1.Ts_control  fcutout=wt1.CurrCont.f_LPF_noise
      settings: SourceProductName=NTNU Power Systems
  Digital first order LPF6 : pwrsysBasic/Digital first order LPF  Commented=on  Ts=wt1.Ts_control  fcutout=wt1.CurrCont.f_LPF_noise
      settings: SourceProductName=NTNU Power Systems
  Divide1 : Product  Inputs=*/
  Enable MSC : Product  Inputs=3
  Enabled : pwrsysBasic/Enabled
      settings: SourceProductName=NTNU Power Systems
  Enabled1 : pwrsysBasic/Enabled
      settings: SourceProductName=NTNU Power Systems
  Gain : Gain  Gain=1/(wt1.Uanp)
  Gain1 : Gain  Gain=1/(wt1.Iap)
  Gain2 : Gain  Gain=1/wt1.Udc
  Gain4 : Gain  Gain=1/wt1.Idc
  Gain5 : Gain  Gain=-wt1.ACVCont.kiq_droop
  Goto21 : Goto  Commented=on  GotoTag=idq_neg
  Goto22 : Goto  Commented=on  GotoTag=vdq_neg
  Idq_Dec_Signs_Fdbk_Ref : pwrsysVICtrl/Idq_Dec_Signs_Fdbk_Ref  Ts=wt1.Ts_control  fn=systemBase.fn  Kp=wt1.CurrContSingle.kp  Ti=wt1.CurrContSingle.Ti  L=wt1.CurrCont.x  PI_max=wt1.CurrCont.PImax  PI_min=wt1.CurrCont.PImin  TrafoPhaseComp=0
      settings: SourceProductName=NTNU Power Systems
  Math Function : Math  Operator=hypot  SaturateOnIntegerOverflow=on
  Mux : Mux  Inputs=2
  NotEqual : RelationalOperator  Operator=~=  OutDataTypeStr=boolean  RndMeth=Nearest
  NotEqual2 : RelationalOperator  Operator=>  OutDataTypeStr=boolean  RndMeth=Nearest
  NotEqual3 : RelationalOperator  Operator=<  OutDataTypeStr=boolean  RndMeth=Nearest
  PI_Std_AntiWindup_HoldUpDown_Backward : pwrsysBasic/PI_Std_AntiWindup_HoldUpDown_Backward  Ts=wt1.Ts_control  Kg=wt1.Qctrl.Kg  Kp=wt1.Qctrl.Kp  Ti=wt1.Qctrl.Ti  outMax=wt1.Qctrl.deltaUmaxPos  outMin=wt1.Qctrl.deltaUmaxNeg
      settings: SourceProductName=NTNU Power Systems
  PLL_pu3 : pwrsysBasic/PLL_pu  fn=systemBase.fn  Ts=wt1.Ts_control  Kp_pll=90  Ki_pll=1200  Kd_pll=0  PLL_ini=60
      settings: SourceProductName=NTNU Power Systems
  Product : Product
  Product1 : Product
  Product2 : Product
  Saturation1 : Saturate  UpperLimit=wt1.DCVCont.PImax  LowerLimit=wt1.DCVCont.PImin
  Saturation2 : Saturate  UpperLimit=1.2  LowerLimit=0.8
  Saturation3 : Saturate  UpperLimit=wt1.Qctrl.Umax  LowerLimit=wt1.Qctrl.Umin
  Scope : Scope  NumInputPorts=4
  Scope1 : Scope
  Scope2 : Scope  NumInputPorts=2
  Selector2 : Selector  IndexMode=Zero-based  InputPortWidth=2  IndexOptions=Index vector (dialog)  Indices=1  OutputSizes=1
  Sum : Sum  Inputs=|++
  Sum1 : Sum  Inputs=+-
  Terminator{1..2,4..10,12} (10 alike) : Terminator
  Uac_Controller : pwrsysVICtrl/Uac_Controller  Ts=wt1.Ts_control  Kg=wt1.ACVCont.kg  Kp=wt1.ACVCont.kp  Ti=wt1.ACVCont.Ti  PI_max=wt1.ACVCont.PImax  PI_min=wt1.ACVCont.PImin
      settings: SourceProductName=NTNU Power Systems
  Udc_Controller : pwrsysVICtrl/Udc_Controller  Ts=wt1.Ts_control  Kp=wt1.DCVContSingle.kp  Ti=wt1.DCVContSingle.Ti  PI_max=wt1.DCVCont.PImax  PI_min=wt1.DCVCont.PImin
      settings: SourceProductName=NTNU Power Systems
  Unit Delay{1,3,7..8} (4 alike) : UnitDelay  InitialCondition=[0 0 0]  SampleTime=wt1.Ts_control
  Unit Delay{2,4..5,9,12..13} (6 alike) : UnitDelay  SampleTime=wt1.Ts_control
  Unit Delay6 : UnitDelay  InitialCondition=1  SampleTime=wt1.Ts_control
  abc_dq_single_notch_dsc_sfunction : pwrsysTransf/abc_dq_single_notch_dsc_sfunction  Ts=wt1.Ts_control  fn=2*systemBase.fn  zeta=wt1.CurrCont.zeta
      settings: SourceProductName=NTNU Power Systems
  dq_to_abc_single_dual : pwrsysVICtrl/dq_to_abc_single_dual  Ts=wt1.Ts_control  Uabp=wt1.Uabp
      settings: SourceProductName=NTNU Power Systems
  pqui_Transd_NoZeroSeq : pwrsysBasic/pqui_Transd_NoZeroSeq  Sn=wt1.Sn  Uanp=col.Uanp  Iap=wt1.Iap*(wt1.Un/col.Un)
      settings: SourceProductName=NTNU Power Systems
  A : PMIOPort  Side=Right
  B : PMIOPort  Port=2  Side=Right
  C : PMIOPort  Port=3  Side=Right
  m : Outport
  wires:
  Divide1/1 -> Enable MSC/3  "Idcref_pu"
  Bus Selector/1 -> Unit Delay1/1  "<LV_Vabc>"
  [idq_pos] -> Selector2/1
  Unit Delay2/1 -> Controlled Current Source1/1
  Gain1/1 -> Bus Creator/8, [iabc]  "Iabc_LV_pu"
  Bus Selector/2 -> Unit Delay3/1  "<LV_Iabc>"
  Gain5/1 -> Add1/2
  Math Function/1 -> Add1/1
  Constant6/1 -> Uac_Controller/7, Uac_Controller/6, Uac_Controller/3, Uac_Controller/4
  Constant5/1 -> Enable MSC/2
  Add1/1 -> Uac_Controller/2  "vac_drooped"
  [mPowerSection] -> Bus Selector/1
  Enable MSC/1 -> Unit Delay2/1  "Idcref_pu"
  Gain/1 -> Bus Creator/7, [vabc]  "Vabc_LV_pu"
  Constant2/1 -> Uac_Controller/5
  Constant8/1 -> Udc_Controller/4, Udc_Controller/5
  NotEqual/1 -> Unit Delay5/1
  [vdc] -> Udc_Controller/1
  Unit Delay5/1 -> Udc_Controller/2
  Saturation1/1 -> NotEqual/2, Mux/1  "idref"
  [idc] -> Add/2
  Udc_Controller/1 -> Add/1
  Add/1 -> NotEqual/1, Saturation1/1
  Constant3/1 -> Udc_Controller/3
  [idq] -> Idq_Dec_Signs_Fdbk_Ref/3
  [Vdc] -> dq_to_abc_single_dual/6
  [wpu] -> Idq_Dec_Signs_Fdbk_Ref/4
  dq_to_abc_single_dual/1 -> Product/2
  [conn] -> Product/1, DCL_LSC_LCL_Trafo_NoSwitching/1
  Saturation2/1 -> Divide1/2
  [Pref] -> Unit Delay9/1  "WT_pref"
  [vdc] -> Saturation2/1
  [wt] -> dq_to_abc_single_dual/7
  Constant10/1 -> abc_dq_single_notch_dsc_sfunction/5
  Bus Selector/5 -> Unit Delay7/1  "<HV_Vabc>"
  Bus Selector/6 -> Unit Delay8/1  "<HV_Iabc>"
  pqui_Transd_NoZeroSeq/1 -> Scope/1, Bus Creator/1  "Pavg_pu"
  pqui_Transd_NoZeroSeq/2 -> Scope/2, [Qavg_pu], Bus Creator/2  "Qavg_pu"
  pqui_Transd_NoZeroSeq/3 -> Scope/3, Bus Creator/3  "Vavg_pu"
  pqui_Transd_NoZeroSeq/4 -> Scope/4, Bus Creator/4  "Iavg_pu"
  Bus Creator/1 -> m/1
  Bus Selector/3 -> Unit Delay6/1  "<INV_Vdc>"
  Gain2/1 -> Scope2/1, Digital first order LPF4/1, Bus Creator/5  "Vdc_pu"
  Gain4/1 -> Scope2/2, [idc], Bus Creator/6  "Idc_pu"
  Bus Selector/4 -> Unit Delay4/1  "<INV_Idc>"
  PLL_pu3/2 -> [wpu]
  PLL_pu3/1 -> [wt]
  Uac_Controller/1 -> Mux/2  "iqref"
  DCL_LSC_LCL_Trafo_NoSwitching/1 -> [mPowerSection]
  Unit Delay1/1 -> Gain/1
  Unit Delay3/1 -> Gain1/1
  Unit Delay4/1 -> Gain4/1
  Unit Delay8/1 -> pqui_Transd_NoZeroSeq/2
  Unit Delay6/1 -> [Vdc], Gain2/1
  Unit Delay7/1 -> pqui_Transd_NoZeroSeq/1
  Unit Delay9/1 -> Divide1/1
  [Vreflim] -> Uac_Controller/1
  abc_dq_single_notch_dsc_sfunction/6 -> Digital first order LPF6/1
  abc_dq_single_notch_dsc_sfunction/5 -> Digital first order LPF5/1
  Selector2/1 -> Gain5/1
  Idq_Dec_Signs_Fdbk_Ref/2 -> Terminator4/1
  [vdq] -> Idq_Dec_Signs_Fdbk_Ref/2
  Constant1/1 -> dq_to_abc_single_dual/2
  Constant7/1 -> dq_to_abc_single_dual/5
  Constant11/1 -> Idq_Dec_Signs_Fdbk_Ref/7, Idq_Dec_Signs_Fdbk_Ref/5
  Constant12/1 -> Idq_Dec_Signs_Fdbk_Ref/8, Idq_Dec_Signs_Fdbk_Ref/9, Idq_Dec_Signs_Fdbk_Ref/10, Idq_Dec_Signs_Fdbk_Ref/6
  Idq_Dec_Signs_Fdbk_Ref/3 -> Terminator5/1
  Idq_Dec_Signs_Fdbk_Ref/4 -> [IdqCtrl]
  [IdqCtrl] -> Bus Creator/9
  Idq_Dec_Signs_Fdbk_Ref/1 -> dq_to_abc_single_dual/1
  [wt] -> abc_dq_single_notch_dsc_sfunction/3
  [wpu] -> abc_dq_single_notch_dsc_sfunction/4
  abc_dq_single_notch_dsc_sfunction/1 -> Digital first order LPF2/1
  [vabc] -> abc_dq_single_notch_dsc_sfunction/1, PLL_pu3/1
  [iabc] -> abc_dq_single_notch_dsc_sfunction/2
  abc_dq_single_notch_dsc_sfunction/3 -> Digital first order LPF1/1
  abc_dq_single_notch_dsc_sfunction/4 -> Digital first order LPF/1
  abc_dq_single_notch_dsc_sfunction/2 -> Digital first order LPF3/1
  Digital first order LPF/1 -> [idq_pos]
  Digital first order LPF1/1 -> [vdq_pos]
  [vdq_pos] -> Demux/1
  Demux/1 -> Math Function/1
  Demux/2 -> Math Function/2
  Digital first order LPF2/1 -> [vdq]
  Digital first order LPF3/1 -> [idq]
  Digital first order LPF4/1 -> [vdc]
  [conn] -> Enable MSC/1
  Pref/1 -> [Pref]
  Mux/1 -> Scope1/1, Idq_Dec_Signs_Fdbk_Ref/1
  Product/1 -> DCL_LSC_LCL_Trafo_NoSwitching/2
  [Vref] -> Sum/2
  Sum/1 -> NotEqual3/1, NotEqual2/1, Saturation3/1
  Saturation3/1 -> NotEqual3/2, NotEqual2/2, [Vreflim]
  [Qavg_pu] -> Sum1/2
  ConsQEn/1 -> Enabled/1
  [QregBlockUp] -> PI_Std_AntiWindup_HoldUpDown_Backward/3
  Constant15/1 -> PI_Std_AntiWindup_HoldUpDown_Backward/2, PI_Std_AntiWindup_HoldUpDown_Backward/4
  [QregBlockDown] -> PI_Std_AntiWindup_HoldUpDown_Backward/5
  Constant18/1 -> PI_Std_AntiWindup_HoldUpDown_Backward/6, PI_Std_AntiWindup_HoldUpDown_Backward/7
  PI_Std_AntiWindup_HoldUpDown_Backward/7 -> Terminator1/1
  PI_Std_AntiWindup_HoldUpDown_Backward/6 -> Terminator6/1
  PI_Std_AntiWindup_HoldUpDown_Backward/5 -> Terminator7/1
  PI_Std_AntiWindup_HoldUpDown_Backward/4 -> Terminator8/1
  PI_Std_AntiWindup_HoldUpDown_Backward/3 -> Terminator9/1
  PI_Std_AntiWindup_HoldUpDown_Backward/2 -> Terminator10/1
  NotEqual2/1 -> Unit Delay12/1
  Unit Delay12/1 -> [QregBlockUp]
  NotEqual3/1 -> Unit Delay13/1
  Unit Delay13/1 -> [QregBlockDown]
  Product2/1 -> Sum/1
  Sum1/1 -> PI_Std_AntiWindup_HoldUpDown_Backward/1
  Enabled/2 -> Terminator12/1
  QavgWF/1 -> Product1/1
  Product1/1 -> Sum1/1
  Enabled/1 -> Product1/2
  Constant13/1 -> [Vref]
  Constant14/1 -> [conn]
  Digital first order LPF5/1 -> Goto22/1
  Digital first order LPF6/1 -> Goto21/1
  Constant9/1 -> dq_to_abc_single_dual/3
  Constant16/1 -> dq_to_abc_single_dual/4
  Enabled1/2 -> Terminator2/1
  PI_Std_AntiWindup_HoldUpDown_Backward/1 -> Product2/2
  Enabled1/1 -> Product2/1
  QregEnable/1 -> Enabled1/1
  connections:
  Controlled Current Source1/RConn1 -- DCL_LSC_LCL_Trafo_NoSwitching/LConn1
  DCL_LSC_LCL_Trafo_NoSwitching/RConn3 -- C/RConn1
  DCL_LSC_LCL_Trafo_NoSwitching/RConn1 -- A/RConn1
  DCL_LSC_LCL_Trafo_NoSwitching/RConn2 -- B/RConn1
  Controlled Current Source1/LConn1 -- DCL_LSC_LCL_Trafo_NoSwitching/LConn2

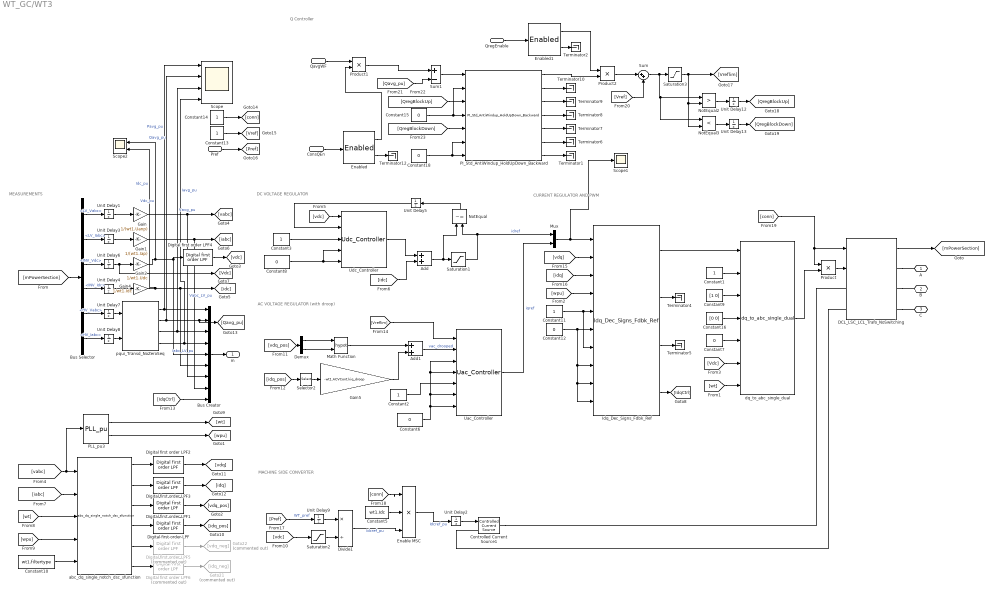
== system WT_GC/WT3 ==
  note: MEASUREMENTS
  note: MACHINE SIDE CONVERTER
  note: AC VOLTAGE REGULATOR (with droop)
  note: DC VOLTAGE REGULATOR
  note: CURRENT REGULATOR AND PWM
  note: Q Controller
  QavgWF : Inport
  ConsQEn : Inport  Port=2
  QregEnable : Inport  Port=3
  Pref : Inport  Port=4
  Add : Sum
  Add1 : Sum
  Bus Creator : BusCreator  Inputs=9
  Bus Selector : BusSelector  OutputSignals=LV_Vabc,LV_Iabc,INV_Vdc,INV_Idc,HV_Vabc,HV_Iabc
  Constant{1..3,11} (4 alike) : Constant  SampleTime=wt1.Ts_control
  Constant10 : Constant  Value=wt1.filtertype  SampleTime=wt1.Ts_control
  Constant{6..8,12} (4 alike) : Constant  Value=0  SampleTime=wt1.Ts_control
  Constant13 : Constant
  Constant14 : Constant
  Constant15 : Constant  Value=0
  Constant16 : Constant  Value=[0 0]  SampleTime=wt1.Ts_control
  Constant18 : Constant  Value=0
  Constant5 : Constant  Value=wt1.Idc  SampleTime=wt1.Ts_control
  Constant9 : Constant  Value=[1 0]  SampleTime=wt1.Ts_control
  Controlled Current Source1 : powerlib/Electrical Sources/Controlled Current Source  Initialize=on  Source_Type=DC  Amplitude=0  Phase=0  Frequency=50  Measurements=None
  DCL_LSC_LCL_Trafo_NoSwitching : pwrsysVSrc/DCL_LSC_LCL_Trafo_NoSwitching  Sn=wt1.Sn  fn=systemBase.fn  Uhv_ab=col.Un  Uab=wt1.Un  lf2=wt1.LCL.l2  rf2=wt1.LCL.r2  Lf1=wt1.LCL.L1  Rf1=wt1.LCL.R1  Cf=wt1.LCL.Cf  Rc=wt1.LCL.Rf  Cdc=wt1.Cdc  Udc0=wt1.Udc  Tsm=wt1.Ts_control  Tstart=wt1.DCVCont.Start
      settings: SourceProductName=NTNU Power Systems
  Demux : Demux  Outputs=2
  Digital first order LPF{,1..4} (5 alike) : pwrsysBasic/Digital first order LPF  Ts=wt1.Ts_control  fcutout=wt1.CurrCont.f_LPF_noise
      settings: SourceProductName=NTNU Power Systems
  Digital first order LPF5 : pwrsysBasic/Digital first order LPF  Commented=on  Ts=wt1.Ts_control  fcutout=wt1.CurrCont.f_LPF_noise
      settings: SourceProductName=NTNU Power Systems
  Digital first order LPF6 : pwrsysBasic/Digital first order LPF  Commented=on  Ts=wt1.Ts_control  fcutout=wt1.CurrCont.f_LPF_noise
      settings: SourceProductName=NTNU Power Systems
  Divide1 : Product  Inputs=*/
  Enable MSC : Product  Inputs=3
  Enabled : pwrsysBasic/Enabled
      settings: SourceProductName=NTNU Power Systems
  Enabled1 : pwrsysBasic/Enabled
      settings: SourceProductName=NTNU Power Systems
  Gain : Gain  Gain=1/(wt1.Uanp)
  Gain1 : Gain  Gain=1/(wt1.Iap)
  Gain2 : Gain  Gain=1/wt1.Udc
  Gain4 : Gain  Gain=1/wt1.Idc
  Gain5 : Gain  Gain=-wt1.ACVCont.kiq_droop
  Goto21 : Goto  Commented=on  GotoTag=idq_neg
  Goto22 : Goto  Commented=on  GotoTag=vdq_neg
  Idq_Dec_Signs_Fdbk_Ref : pwrsysVICtrl/Idq_Dec_Signs_Fdbk_Ref  Ts=wt1.Ts_control  fn=systemBase.fn  Kp=wt1.CurrContSingle.kp  Ti=wt1.CurrContSingle.Ti  L=wt1.CurrCont.x  PI_max=wt1.CurrCont.PImax  PI_min=wt1.CurrCont.PImin  TrafoPhaseComp=0
      settings: SourceProductName=NTNU Power Systems
  Math Function : Math  Operator=hypot  SaturateOnIntegerOverflow=on
  Mux : Mux  Inputs=2
  NotEqual : RelationalOperator  Operator=~=  OutDataTypeStr=boolean  RndMeth=Nearest
  NotEqual2 : RelationalOperator  Operator=>  OutDataTypeStr=boolean  RndMeth=Nearest
  NotEqual3 : RelationalOperator  Operator=<  OutDataTypeStr=boolean  RndMeth=Nearest
  PI_Std_AntiWindup_HoldUpDown_Backward : pwrsysBasic/PI_Std_AntiWindup_HoldUpDown_Backward  Ts=wt1.Ts_control  Kg=wt1.Qctrl.Kg  Kp=wt1.Qctrl.Kp  Ti=wt1.Qctrl.Ti  outMax=wt1.Qctrl.deltaUmaxPos  outMin=wt1.Qctrl.deltaUmaxNeg
      settings: SourceProductName=NTNU Power Systems
  PLL_pu3 : pwrsysBasic/PLL_pu  fn=systemBase.fn  Ts=wt1.Ts_control  Kp_pll=90  Ki_pll=1200  Kd_pll=0  PLL_ini=60
      settings: SourceProductName=NTNU Power Systems
  Product : Product
  Product1 : Product
  Product2 : Product
  Saturation1 : Saturate  UpperLimit=wt1.DCVCont.PImax  LowerLimit=wt1.DCVCont.PImin
  Saturation2 : Saturate  UpperLimit=1.2  LowerLimit=0.8
  Saturation3 : Saturate  UpperLimit=wt1.Qctrl.Umax  LowerLimit=wt1.Qctrl.Umin
  Scope : Scope  NumInputPorts=4
  Scope1 : Scope
  Scope2 : Scope  NumInputPorts=2
  Selector2 : Selector  IndexMode=Zero-based  InputPortWidth=2  IndexOptions=Index vector (dialog)  Indices=1  OutputSizes=1
  Sum : Sum  Inputs=|++
  Sum1 : Sum  Inputs=+-
  Terminator{1..2,4..10,12} (10 alike) : Terminator
  Uac_Controller : pwrsysVICtrl/Uac_Controller  Ts=wt1.Ts_control  Kg=wt1.ACVCont.kg  Kp=wt1.ACVCont.kp  Ti=wt1.ACVCont.Ti  PI_max=wt1.ACVCont.PImax  PI_min=wt1.ACVCont.PImin
      settings: SourceProductName=NTNU Power Systems
  Udc_Controller : pwrsysVICtrl/Udc_Controller  Ts=wt1.Ts_control  Kp=wt1.DCVContSingle.kp  Ti=wt1.DCVContSingle.Ti  PI_max=wt1.DCVCont.PImax  PI_min=wt1.DCVCont.PImin
      settings: SourceProductName=NTNU Power Systems
  Unit Delay{1,3,7..8} (4 alike) : UnitDelay  InitialCondition=[0 0 0]  SampleTime=wt1.Ts_control
  Unit Delay{2,4..5,9,12..13} (6 alike) : UnitDelay  SampleTime=wt1.Ts_control
  Unit Delay6 : UnitDelay  InitialCondition=1  SampleTime=wt1.Ts_control
  abc_dq_single_notch_dsc_sfunction : pwrsysTransf/abc_dq_single_notch_dsc_sfunction  Ts=wt1.Ts_control  fn=2*systemBase.fn  zeta=wt1.CurrCont.zeta
      settings: SourceProductName=NTNU Power Systems
  dq_to_abc_single_dual : pwrsysVICtrl/dq_to_abc_single_dual  Ts=wt1.Ts_control  Uabp=wt1.Uabp
      settings: SourceProductName=NTNU Power Systems
  pqui_Transd_NoZeroSeq : pwrsysBasic/pqui_Transd_NoZeroSeq  Sn=wt1.Sn  Uanp=col.Uanp  Iap=wt1.Iap*(wt1.Un/col.Un)
      settings: SourceProductName=NTNU Power Systems
  A : PMIOPort  Side=Right
  B : PMIOPort  Port=2  Side=Right
  C : PMIOPort  Port=3  Side=Right
  m : Outport
  wires:
  Divide1/1 -> Enable MSC/3  "Idcref_pu"
  Bus Selector/1 -> Unit Delay1/1  "<LV_Vabc>"
  [idq_pos] -> Selector2/1
  Unit Delay2/1 -> Controlled Current Source1/1
  Gain1/1 -> Bus Creator/8, [iabc]  "Iabc_LV_pu"
  Bus Selector/2 -> Unit Delay3/1  "<LV_Iabc>"
  Gain5/1 -> Add1/2
  Math Function/1 -> Add1/1
  Constant6/1 -> Uac_Controller/7, Uac_Controller/6, Uac_Controller/3, Uac_Controller/4
  Constant5/1 -> Enable MSC/2
  Add1/1 -> Uac_Controller/2  "vac_drooped"
  [mPowerSection] -> Bus Selector/1
  Enable MSC/1 -> Unit Delay2/1  "Idcref_pu"
  Gain/1 -> Bus Creator/7, [vabc]  "Vabc_LV_pu"
  Constant2/1 -> Uac_Controller/5
  Constant8/1 -> Udc_Controller/4, Udc_Controller/5
  NotEqual/1 -> Unit Delay5/1
  [vdc] -> Udc_Controller/1
  Unit Delay5/1 -> Udc_Controller/2
  Saturation1/1 -> NotEqual/2, Mux/1  "idref"
  [idc] -> Add/2
  Udc_Controller/1 -> Add/1
  Add/1 -> NotEqual/1, Saturation1/1
  Constant3/1 -> Udc_Controller/3
  [idq] -> Idq_Dec_Signs_Fdbk_Ref/3
  [Vdc] -> dq_to_abc_single_dual/6
  [wpu] -> Idq_Dec_Signs_Fdbk_Ref/4
  dq_to_abc_single_dual/1 -> Product/2
  [conn] -> Product/1, DCL_LSC_LCL_Trafo_NoSwitching/1
  Saturation2/1 -> Divide1/2
  [Pref] -> Unit Delay9/1  "WT_pref"
  [vdc] -> Saturation2/1
  [wt] -> dq_to_abc_single_dual/7
  Constant10/1 -> abc_dq_single_notch_dsc_sfunction/5
  Bus Selector/5 -> Unit Delay7/1  "<HV_Vabc>"
  Bus Selector/6 -> Unit Delay8/1  "<HV_Iabc>"
  pqui_Transd_NoZeroSeq/1 -> Scope/1, Bus Creator/1  "Pavg_pu"
  pqui_Transd_NoZeroSeq/2 -> Scope/2, [Qavg_pu], Bus Creator/2  "Qavg_pu"
  pqui_Transd_NoZeroSeq/3 -> Scope/3, Bus Creator/3  "Vavg_pu"
  pqui_Transd_NoZeroSeq/4 -> Scope/4, Bus Creator/4  "Iavg_pu"
  Bus Creator/1 -> m/1
  Bus Selector/3 -> Unit Delay6/1  "<INV_Vdc>"
  Gain2/1 -> Scope2/1, Digital first order LPF4/1, Bus Creator/5  "Vdc_pu"
  Gain4/1 -> Scope2/2, [idc], Bus Creator/6  "Idc_pu"
  Bus Selector/4 -> Unit Delay4/1  "<INV_Idc>"
  PLL_pu3/2 -> [wpu]
  PLL_pu3/1 -> [wt]
  Uac_Controller/1 -> Mux/2  "iqref"
  DCL_LSC_LCL_Trafo_NoSwitching/1 -> [mPowerSection]
  Unit Delay1/1 -> Gain/1
  Unit Delay3/1 -> Gain1/1
  Unit Delay4/1 -> Gain4/1
  Unit Delay8/1 -> pqui_Transd_NoZeroSeq/2
  Unit Delay6/1 -> [Vdc], Gain2/1
  Unit Delay7/1 -> pqui_Transd_NoZeroSeq/1
  Unit Delay9/1 -> Divide1/1
  [Vreflim] -> Uac_Controller/1
  abc_dq_single_notch_dsc_sfunction/6 -> Digital first order LPF6/1
  abc_dq_single_notch_dsc_sfunction/5 -> Digital first order LPF5/1
  Selector2/1 -> Gain5/1
  Idq_Dec_Signs_Fdbk_Ref/2 -> Terminator4/1
  [vdq] -> Idq_Dec_Signs_Fdbk_Ref/2
  Constant1/1 -> dq_to_abc_single_dual/2
  Constant7/1 -> dq_to_abc_single_dual/5
  Constant11/1 -> Idq_Dec_Signs_Fdbk_Ref/7, Idq_Dec_Signs_Fdbk_Ref/5
  Constant12/1 -> Idq_Dec_Signs_Fdbk_Ref/8, Idq_Dec_Signs_Fdbk_Ref/9, Idq_Dec_Signs_Fdbk_Ref/10, Idq_Dec_Signs_Fdbk_Ref/6
  Idq_Dec_Signs_Fdbk_Ref/3 -> Terminator5/1
  Idq_Dec_Signs_Fdbk_Ref/4 -> [IdqCtrl]
  [IdqCtrl] -> Bus Creator/9
  Idq_Dec_Signs_Fdbk_Ref/1 -> dq_to_abc_single_dual/1
  [wt] -> abc_dq_single_notch_dsc_sfunction/3
  [wpu] -> abc_dq_single_notch_dsc_sfunction/4
  abc_dq_single_notch_dsc_sfunction/1 -> Digital first order LPF2/1
  [vabc] -> abc_dq_single_notch_dsc_sfunction/1, PLL_pu3/1
  [iabc] -> abc_dq_single_notch_dsc_sfunction/2
  abc_dq_single_notch_dsc_sfunction/3 -> Digital first order LPF1/1
  abc_dq_single_notch_dsc_sfunction/4 -> Digital first order LPF/1
  abc_dq_single_notch_dsc_sfunction/2 -> Digital first order LPF3/1
  Digital first order LPF/1 -> [idq_pos]
  Digital first order LPF1/1 -> [vdq_pos]
  [vdq_pos] -> Demux/1
  Demux/1 -> Math Function/1
  Demux/2 -> Math Function/2
  Digital first order LPF2/1 -> [vdq]
  Digital first order LPF3/1 -> [idq]
  Digital first order LPF4/1 -> [vdc]
  [conn] -> Enable MSC/1
  Pref/1 -> [Pref]
  Mux/1 -> Scope1/1, Idq_Dec_Signs_Fdbk_Ref/1
  Product/1 -> DCL_LSC_LCL_Trafo_NoSwitching/2
  [Vref] -> Sum/2
  Sum/1 -> NotEqual3/1, NotEqual2/1, Saturation3/1
  Saturation3/1 -> NotEqual3/2, NotEqual2/2, [Vreflim]
  [Qavg_pu] -> Sum1/2
  ConsQEn/1 -> Enabled/1
  [QregBlockUp] -> PI_Std_AntiWindup_HoldUpDown_Backward/3
  Constant15/1 -> PI_Std_AntiWindup_HoldUpDown_Backward/2, PI_Std_AntiWindup_HoldUpDown_Backward/4
  [QregBlockDown] -> PI_Std_AntiWindup_HoldUpDown_Backward/5
  Constant18/1 -> PI_Std_AntiWindup_HoldUpDown_Backward/6, PI_Std_AntiWindup_HoldUpDown_Backward/7
  PI_Std_AntiWindup_HoldUpDown_Backward/7 -> Terminator1/1
  PI_Std_AntiWindup_HoldUpDown_Backward/6 -> Terminator6/1
  PI_Std_AntiWindup_HoldUpDown_Backward/5 -> Terminator7/1
  PI_Std_AntiWindup_HoldUpDown_Backward/4 -> Terminator8/1
  PI_Std_AntiWindup_HoldUpDown_Backward/3 -> Terminator9/1
  PI_Std_AntiWindup_HoldUpDown_Backward/2 -> Terminator10/1
  NotEqual2/1 -> Unit Delay12/1
  Unit Delay12/1 -> [QregBlockUp]
  NotEqual3/1 -> Unit Delay13/1
  Unit Delay13/1 -> [QregBlockDown]
  Product2/1 -> Sum/1
  Sum1/1 -> PI_Std_AntiWindup_HoldUpDown_Backward/1
  Enabled/2 -> Terminator12/1
  QavgWF/1 -> Product1/1
  Product1/1 -> Sum1/1
  Enabled/1 -> Product1/2
  Constant13/1 -> [Vref]
  Constant14/1 -> [conn]
  Digital first order LPF5/1 -> Goto22/1
  Digital first order LPF6/1 -> Goto21/1
  Constant9/1 -> dq_to_abc_single_dual/3
  Constant16/1 -> dq_to_abc_single_dual/4
  Enabled1/2 -> Terminator2/1
  PI_Std_AntiWindup_HoldUpDown_Backward/1 -> Product2/2
  Enabled1/1 -> Product2/1
  QregEnable/1 -> Enabled1/1
  connections:
  Controlled Current Source1/RConn1 -- DCL_LSC_LCL_Trafo_NoSwitching/LConn1
  DCL_LSC_LCL_Trafo_NoSwitching/RConn3 -- C/RConn1
  DCL_LSC_LCL_Trafo_NoSwitching/RConn1 -- A/RConn1
  DCL_LSC_LCL_Trafo_NoSwitching/RConn2 -- B/RConn1
  Controlled Current Source1/LConn1 -- DCL_LSC_LCL_Trafo_NoSwitching/LConn2
